simulink model "mips"  (R2012b)
settings: Solver=ode45  SolverMode=SingleTasking  StartTime=0.0  StopTime=100  RelTol=1e-3
libraries: xbsIndex_r4 x13
settings Model: Creator=craig  LastModifiedBy=dsho996
settings DataIOCC: SignalLoggingSaveFormat=ModelDataLogs
settings OptimizationCC: BlockReduction=off  BooleanDataType=off
settings DebuggingCC: SaveWithParameterizedLinksMsg=none  SignalResolutionControl=TryResolveAllWithWarning  SolverPrmCheckMsg=none  MultiTaskDSMMsg=warning  MultiTaskCondExecSysMsg=none  FcnCallInpInsideContextMsg=EnableAllAsWarning  StrictBusMsg=None
settings HardwareCC: TargetIntDivRoundTo=Zero  TargetEndianess=LittleEndian  TargetHWDeviceType=MATLAB Host  ProdEqTarget=off
settings RTWCC: IncludeERTFirstTime=on

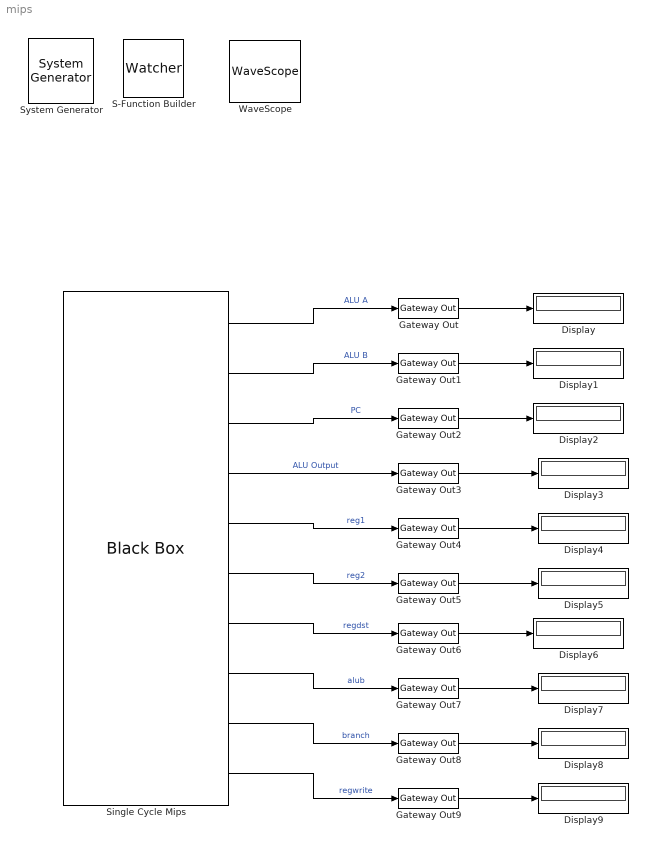
== system mips ==
  " System Generator" : xbsIndex_r4/ System Generator  Tag=genX  xilinxfamily=Kintex7  part=xc7k325t  speed=-3  package=fbg676  synthesis_tool=XST  clock_wrapper=Clock Enables  directory=./netlist  proj_type=Project Navigator  Synth_file=XST Defaults  Impl_file=ISE Defaults  testbench=off  simulink_period=1  sysclk_period=10  dcm_input_clock_period=10  incr_netlist=off  trim_vbits=Everywhere in SubSystem  dbl_ovrd=According to Block Masks  core_generation=According to Block Masks  run_coregen=off  deprecated_control=off  eval_field=0  block_type=sysgen
  Display{,1..9} (10 alike) : Display
  Gateway Out{,1..9} (10 alike) : xbsIndex_r4/Gateway Out  inherit_from_input=off  hdl_port=on  timing_constraint=None  locs_specified=off  LOCs={}  UseAsDAC=off  DACChannel='1'  block_type=gatewayout
  S-Function Builder : S-Function  FunctionName=Watcher  SFunctionModules=Watcher_wrapper NotifyServer RecordLookup  EnableBusSupport=off  mask(S-Function Builder){}
      mask help: Simulink:masks:SFunctionBuilder_MD
      mask init:
      | val = [[.9  0.75 0.75 1 1 .9 .9 1]',[1 1 0.75 0.75 .9 .9 1 .9]'];try , sys = get_param(gcb,'SfunBuilderFcnName');if isempty(sys), sys = get_param(gcb,'FunctionName'); end,catch, sys = get_param(gcb,'FunctionName'); end
      settings: CopyFcn=set_param(gcbh,'LinkStatus','none')  PreSaveFcn=try, set_param(gcb,'FunctionName','Watcher'), end  OpenFcn=sfunctionwizard(gcbh)
      mask Display: plot(val(:,1),val(:,2)),disp(sys), port_label('input',1,'ALLOW_ZERO_PORTS'), port_label('output',1,'ALLOW_ZERO_PORTS')
  Single Cycle Mips : xbsIndex_r4/Black Box  init_code=mips_top_config  sim_method=ISE Simulator  verbose=off  block_type=blackbox2
  WaveScope : xbsIndex_r4/WaveScope  block_type=wavescope
  wires:
  Gateway Out/1 -> Display/1
  Gateway Out1/1 -> Display1/1
  Gateway Out2/1 -> Display2/1
  Gateway Out3/1 -> Display3/1
  Gateway Out4/1 -> Display4/1
  Gateway Out5/1 -> Display5/1
  Single Cycle Mips/1 -> Gateway Out/1  "ALU A"
  Single Cycle Mips/2 -> Gateway Out1/1  "ALU B"
  Single Cycle Mips/3 -> Gateway Out2/1  "PC"
  Single Cycle Mips/4 -> Gateway Out3/1  "ALU Output"
  Single Cycle Mips/5 -> Gateway Out4/1  "reg1"
  Single Cycle Mips/6 -> Gateway Out5/1  "reg2"
  Gateway Out6/1 -> Display6/1
  Gateway Out7/1 -> Display7/1
  Gateway Out8/1 -> Display8/1
  Gateway Out9/1 -> Display9/1
  Single Cycle Mips/7 -> Gateway Out6/1  "regdst"
  Single Cycle Mips/8 -> Gateway Out7/1  "alub"
  Single Cycle Mips/9 -> Gateway Out8/1  "branch"
  Single Cycle Mips/10 -> Gateway Out9/1  "regwrite"
